simulink model "modelo_fisico_v18"  (R2021a)
settings: Solver=ode23  StartTime=0.0  StopTime=inf  MinStep=1e-4
values from neighbouring files (symbols this model uses):
  a_hMax = 0.75    [Datos_ProyectoGlobal_AyCD_Cantu_LagoTejo.m]    (also in Datos_v18.m; PID_calculado.mat)
  a_tMax = 0.8    [Datos_ProyectoGlobal_AyCD_Cantu_LagoTejo.m]    (also in Datos_v18.m; PID_calculado.mat)
  b_cx = 1e6    (= 1000000)    [Datos_ProyectoGlobal_AyCD_Cantu_LagoTejo.m]    (also in Datos_v18.m; PID_calculado.mat)
  b_cy = 1e7    (= 10000000)    [Datos_ProyectoGlobal_AyCD_Cantu_LagoTejo.m]    (also in Datos_v18.m; PID_calculado.mat)
  b_eq_h = ((b_hd + b_hm*(i_h^2))*2/(r_hd^2))    (= 31004.4444444)    [Datos_ProyectoGlobal_AyCD_Cantu_LagoTejo.m]    (also in Datos_v18.m; PID_calculado.mat)
  b_eq_t = ((b_td + b_tm*(i_t^2))/(r_td^2))    (= 21607.2)    [Datos_ProyectoGlobal_AyCD_Cantu_LagoTejo.m]    (also in Datos_v18.m; PID_calculado.mat)
  b_hb = 1e8    (= 100000000)    [Datos_ProyectoGlobal_AyCD_Cantu_LagoTejo.m]    (also in Datos_v18.m; PID_calculado.mat)
  b_hEb = 2.2e9    (= 2200000000)    [Datos_ProyectoGlobal_AyCD_Cantu_LagoTejo.m]    (also in Datos_v18.m; PID_calculado.mat)
  b_t = 90    [Datos_ProyectoGlobal_AyCD_Cantu_LagoTejo.m]    (also in Datos_v18.m; PID_calculado.mat)
  b_tb = 5e6    (= 5000000)    [Datos_ProyectoGlobal_AyCD_Cantu_LagoTejo.m]    (also in Datos_v18.m; PID_calculado.mat)
  b_tw = 3e3    (= 3000)    [Datos_ProyectoGlobal_AyCD_Cantu_LagoTejo.m]    (also in Datos_v18.m; PID_calculado.mat)
  b_wu = 150    [Datos_ProyectoGlobal_AyCD_Cantu_LagoTejo.m]    (also in Datos_v18.m; PID_calculado.mat)
  bah = M_eq_h*n_h*omega_h    [PID_Izaje_B.m]    (also in PID_calculado.mat = 387555.555556)
  bat = M_eq_t*n_t*omega_t    [PID_Carro_B.m]    (also in PID_calculado.mat = 270090)
  CI_h = 5    [Datos_ProyectoGlobal_AyCD_Cantu_LagoTejo.m]    (also in Datos_v18.m; PID_calculado.mat)
  CI_t = -16.25    [Datos_ProyectoGlobal_AyCD_Cantu_LagoTejo.m]    (also in Datos_v18.m; PID_calculado.mat)
  d_t = 1e-3    (= 0.001)    [Datos_ProyectoGlobal_AyCD_Cantu_LagoTejo.m]    (also in Datos_v18.m; PID_calculado.mat)
  g = 9.80665    [Datos_ProyectoGlobal_AyCD_Cantu_LagoTejo.m]    (also in Datos_v18.m; PID_calculado.mat)
  H_c = 2.5    [Datos_ProyectoGlobal_AyCD_Cantu_LagoTejo.m]    (also in Datos_v18.m; PID_calculado.mat)
  i_h = 22    [Datos_ProyectoGlobal_AyCD_Cantu_LagoTejo.m]    (also in Datos_v18.m; PID_calculado.mat)
  i_t = 30    [Datos_ProyectoGlobal_AyCD_Cantu_LagoTejo.m]    (also in Datos_v18.m; PID_calculado.mat)
  k_cy = 1.8e9    (= 1800000000)    [Datos_ProyectoGlobal_AyCD_Cantu_LagoTejo.m]    (also in Datos_v18.m; PID_calculado.mat)
  k_tw = 4.8e5    (= 480000)    [Datos_ProyectoGlobal_AyCD_Cantu_LagoTejo.m]    (also in Datos_v18.m; PID_calculado.mat)
  k_wu = 2.36e8    (= 236000000)    [Datos_ProyectoGlobal_AyCD_Cantu_LagoTejo.m]    (also in Datos_v18.m; PID_calculado.mat)
  Kd_bal = [-2.22044604925e-16 2.22044604925e-16 2.22044604925e-16 0 0 0 0 0 -2.22044604925e-16 0 2.22044604925e-16 -2.22044604925e-16 ... (296091 elements, 501x591)]    [Kp_Kd_balanceo.mat]    (also in PD_Balanceo.m = zeros(length(ML),length(L)))
  Kp_bal = [5.11381136401 5.1081388039 5.10248507909 5.09685008556 5.09123372013 5.08563588037 5.08005646467 5.07449537218 5.06895250283 5.06342775732 5.05792103709 5.05243224433 ... (296091 elements, 501x591)]    [Kp_Kd_balanceo.mat]    (also in PD_Balanceo.m = Kd_bal)
  ksah = M_eq_h*n_h*(omega_h^2)    [PID_Izaje_B.m]    (also in PID_calculado.mat = 922348.374575)
  ksat = M_eq_t*n_t*(omega_t^2)    [PID_Carro_B.m]    (also in PID_calculado.mat = 972648.108)
  ksiah = M_eq_h*n_h*(omega_h^3)    [PID_Izaje_B.m]    (also in PID_calculado.mat = 2195108.57705)
  ksiat = M_eq_t*n_t*(omega_t^3)    [PID_Carro_B.m]    (also in PID_calculado.mat = 3502700.36653)
  lim_xDer = 50    [Datos_ProyectoGlobal_AyCD_Cantu_LagoTejo.m]    (also in Datos_v18.m; PID_calculado.mat)
  lim_xDer_ult = 51    [Datos_ProyectoGlobal_AyCD_Cantu_LagoTejo.m]    (also in Datos_v18.m; PID_calculado.mat)
  lim_xIzq = -30    [Datos_ProyectoGlobal_AyCD_Cantu_LagoTejo.m]    (also in Datos_v18.m; PID_calculado.mat)
  lim_xIzq_ult = -31    [Datos_ProyectoGlobal_AyCD_Cantu_LagoTejo.m]    (also in Datos_v18.m; PID_calculado.mat)
  lim_yInf = -20    [Datos_ProyectoGlobal_AyCD_Cantu_LagoTejo.m]    (also in Datos_v18.m; PID_calculado.mat)
  lim_yInf_ult = -21    [Datos_ProyectoGlobal_AyCD_Cantu_LagoTejo.m]    (also in Datos_v18.m; PID_calculado.mat)
  lim_ySup = 40    [Datos_ProyectoGlobal_AyCD_Cantu_LagoTejo.m]    (also in Datos_v18.m; PID_calculado.mat)
  lim_ySup_ult = 41    [Datos_ProyectoGlobal_AyCD_Cantu_LagoTejo.m]    (also in Datos_v18.m; PID_calculado.mat)
  M_cMax = 50000    [Datos_ProyectoGlobal_AyCD_Cantu_LagoTejo.m]    (also in Datos_v18.m; PID_calculado.mat)
  M_cMin = 2000    [Datos_ProyectoGlobal_AyCD_Cantu_LagoTejo.m]    (also in Datos_v18.m; PID_calculado.mat)
  M_eq_h = (J_hd_hEb+J_hm_hb*i_h^2)*2/r_hd^2    (= 65137.7777778)    [Datos_ProyectoGlobal_AyCD_Cantu_LagoTejo.m]    (also in Datos_v18.m; PID_calculado.mat)
  M_eq_t = ((J_td + J_tm_tb*(i_t^2))/(r_td^2))    (= 30000)    [Datos_ProyectoGlobal_AyCD_Cantu_LagoTejo.m]    (also in Datos_v18.m; PID_calculado.mat)
  M_l_max = 32500    [Datos_ProyectoGlobal_AyCD_Cantu_LagoTejo.m]    (also in Datos_v18.m; PID_calculado.mat)
  M_l_nom = 65000    [Datos_ProyectoGlobal_AyCD_Cantu_LagoTejo.m]    (also in Datos_v18.m; PID_calculado.mat)
  M_s = 15000    [Datos_ProyectoGlobal_AyCD_Cantu_LagoTejo.m]    (also in Datos_v18.m; PID_calculado.mat)
  M_t = 30000    [Datos_ProyectoGlobal_AyCD_Cantu_LagoTejo.m]    (also in Datos_v18.m; PID_calculado.mat)
  P_h_nom = 956.15e3    (= 956150)    [Datos_ProyectoGlobal_AyCD_Cantu_LagoTejo.m]    (also in Datos_v18.m; PID_calculado.mat)
  r_hd = 0.75    [Datos_ProyectoGlobal_AyCD_Cantu_LagoTejo.m]    (also in Datos_v18.m; PID_calculado.mat)
  r_td = 0.5    [Datos_ProyectoGlobal_AyCD_Cantu_LagoTejo.m]    (also in Datos_v18.m; PID_calculado.mat)
  T_hbMax = 5e4    (= 50000)    [Datos_ProyectoGlobal_AyCD_Cantu_LagoTejo.m]    (also in Datos_v18.m; PID_calculado.mat)
  T_hEbMax = 1.1e6    (= 1100000)    [Datos_ProyectoGlobal_AyCD_Cantu_LagoTejo.m]    (also in Datos_v18.m; PID_calculado.mat)
  T_hmMax = 2e4    (= 20000)    [Datos_ProyectoGlobal_AyCD_Cantu_LagoTejo.m]    (also in Datos_v18.m; PID_calculado.mat)
  T_tbMax = 5e3    (= 5000)    [Datos_ProyectoGlobal_AyCD_Cantu_LagoTejo.m]    (also in Datos_v18.m; PID_calculado.mat)
  T_tmMax = 3e3    (= 3000)    [Datos_ProyectoGlobal_AyCD_Cantu_LagoTejo.m]    (also in Datos_v18.m; PID_calculado.mat)
  tau_hm = 1e-3    (= 0.001)    [Datos_ProyectoGlobal_AyCD_Cantu_LagoTejo.m]    (also in Datos_v18.m; PID_calculado.mat)
  tau_tm = 1e-3    (= 0.001)    [Datos_ProyectoGlobal_AyCD_Cantu_LagoTejo.m]    (also in Datos_v18.m; PID_calculado.mat)
  v_hMax_0 = 3    [Datos_ProyectoGlobal_AyCD_Cantu_LagoTejo.m]    (also in Datos_v18.m; PID_calculado.mat)
  v_hMax_l = 1.5    [Datos_ProyectoGlobal_AyCD_Cantu_LagoTejo.m]    (also in Datos_v18.m; PID_calculado.mat)
  v_tMax = 4    [Datos_ProyectoGlobal_AyCD_Cantu_LagoTejo.m]    (also in Datos_v18.m; PID_calculado.mat)
  xc = [-28.75 -26.25 -23.75 -21.25 -18.75 -16.25 -13.75 -11.25 -8.75 -6.25 -3.75 -1.25 ... (32 elements, 1x32)]    [PID_calculado.mat]    (also in Perfil_Carga.m = -30+1.25:2.5:50-1.25)
  Y_sb = 15    [Datos_ProyectoGlobal_AyCD_Cantu_LagoTejo.m]    (also in Datos_v18.m; PID_calculado.mat)
  Y_t0 = 45    [Datos_ProyectoGlobal_AyCD_Cantu_LagoTejo.m]    (also in Datos_v18.m; PID_calculado.mat)
  yc = [0 0 0 2.5 0 2.5 0 2.5 0 0 0 0 ... (32 elements, 1x32)]    [PID_calculado.mat]    (also in Perfil_Carga.m = yc2)
undefined symbols (not defined in the file or in its folder): bcx, bcy, Cond_Ini_h, Cond_Ini_t, Kcy
libraries: simulink x13
(part 1 of 3)
settings Model: SimulationMode=accelerator  Creator=Maxi  LastModifiedBy=maxim
settings SolverCC: InitialStep=1e-3  MaxConsecutiveZCs=10000  MaxConsecutiveMinStep=10000000  ZeroCrossAlgorithm=Adaptive  AlgebraicLoopSolver=TrustRegion
settings DebuggingCC: AlgebraicLoopMsg=none  MaskedZcDiagnostic=none  IgnoredZcDiagnostic=none  SFUnusedDataAndEventsDiag=none  UnderSpecifiedDimensionMsg=warning
settings RTWCC: DLArmComputeVersion=20.02.1

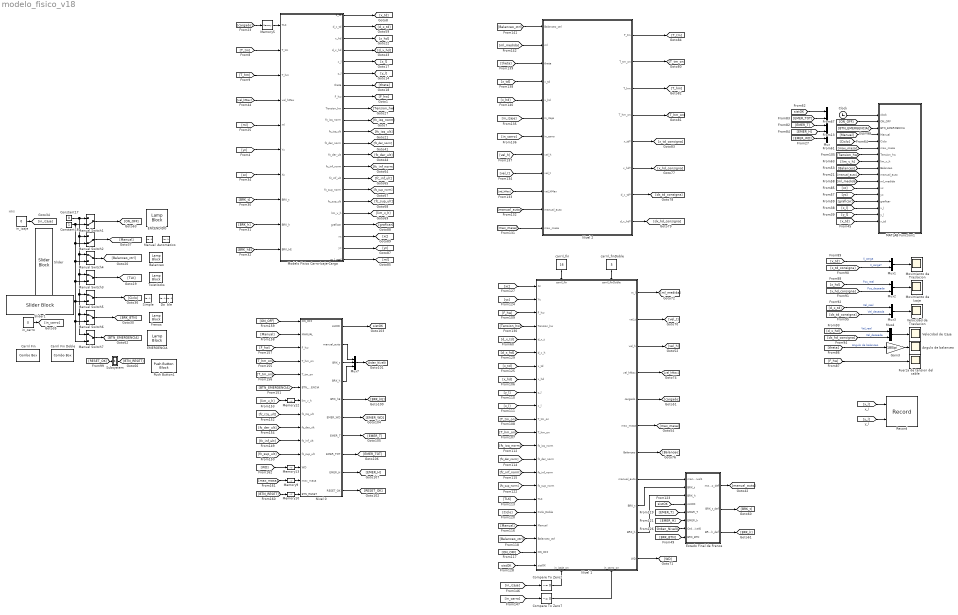
== system modelo_fisico_v18 ==
  note: HMI
  "  Do" : LampBlock  LabelPosition=Hide
  Angulo de balanceo : Scope
  Automático : LampBlock  LabelPosition=Hide
  Balanceo : LampBlock  LabelPosition=Hide
  Carril Fin : ComboBox  LabelPosition=Hide  SelectedLabel=16
      settings: Values={{'1', '2', '3', '4', '5', '6', '7', '8', '9', '10', '11', '12', '13', '14', '15', '16', '17', '18'}, [1 2 3 4 5 6 7 8 9 10 11 12 13 14 15 16 17 18]}
  Carril Fin Doble : ComboBox  LabelPosition=Hide  SelectedLabel=5
      settings: Values={{'1', '2', '3', '4', '5', '6', '7', '8', '9', '10', '11', '12', '13', '14', '15', '16', '17', '18'}, [1 2 3 4 5 6 7 8 9 10 11 12 13 14 15 16 17 18]}
  Clock : Clock
  Compare To Zero2 : simulink/Logic and Bit Operations/Compare To Zero  relop=~=  OutDataTypeStr=boolean
  Compare To Zero7 : simulink/Logic and Bit Operations/Compare To Zero  relop=~=  OutDataTypeStr=boolean
  Constant17 : Constant  Value=0
  Constant18 : Constant
  EMERGENCIA : LampBlock  LabelPosition=Hide
  ENCENDIDO : LampBlock  LabelPosition=Hide
  Estado Final de Frenos : Subsystem
  Frenos : LampBlock  LabelPosition=Hide
  Fuerza de tension del cable : Scope
  Gain3 : Gain  Gain=180/pi
  MATLAB Function1 : MATLAB Function  TreatAsAtomicUnit=on
  Manual : LampBlock  LabelPosition=Hide
  Manual Switch1 : ManualSwitch  CurrentSetting=0
  Manual Switch2 : ManualSwitch  CurrentSetting=0
  Manual Switch{3..7} (5 alike) : ManualSwitch
  Memory{5,9..10,12..13} (5 alike) : Memory
  Modelo Fisico Carro-Izaje-Carga : Subsystem
  Movimiento de Izaje : Scope
  Movimiento de Traslacion : Scope
  Mux : Mux  Inputs=5
  Mux{1..4} (4 alike) : Mux  Inputs=2
  Mux7 : Mux  Inputs=3
  Nivel 0 : Stateflow chart  TreatAsAtomicUnit=on
      settings: PortSchema="{\"entries\":[{\"content\":{\"sides\":[{\"content\":{\"connectorIds\":[\"In6\",\"In7\",\"In5\",\"In2\",\"In1\",\"In3\",\"In4\",\"In8\",\"In9\",\"In10\",\"In11\",\"In12\",\"In13\",\"In14\"]},\"type\":\"ConnectorPlacement.EquallySpacedRectSide\",\"uuid\":\"e3679c49-321c-4245-9f4d-6b72d70eef8d\"},{\"content\":{\"connectorIds\":[\"Out1\",\"Out3\",\"Out5\",\"Out4\",\"Out2\",\"Out6\",\"Out7\",\"Out8\",\"Out9\",\"Out10\"],\"side\":\"RIGHT\"},\"type\":\"ConnectorPlacement.EquallySpacedRectSide\",\"uuid\":\"16418e5e-e28d-455d-933a-43b8d78ab460\"},{\"content\":{\"side\":\"TOP\"},\"type\":\"ConnectorPlacement.EquallySpacedRectSide\",\"uuid\":\"c85d7e80-ad5f-4217-ba10-6288ee566bb8\"}]},\"type\":\"ConnectorPlacement.EquallySpacedConnector\",\"uuid\":\"c38c6e76-5322-4b57-8473-560e5b1141d3\"}],\"packageUris\":[\"http://schema.mathworks.com/mf0/Connector/R2020b\"],\"version\":\"1.0\"}"
  Nivel 1 : Stateflow chart  TreatAsAtomicUnit=on
      settings: PortSchema="{\"entries\":[{\"content\":{\"sides\":[{\"content\":{\"connectorIds\":[\"In23\",\"In22\",\"In12\",\"In24\",\"In21\",\"In20\",\"In10\",\"In11\",\"In19\",\"In5\",\"In9\",\"In4\",\"In15\",\"In16\",\"In17\",\"In18\",\"In3\",\"In14\",\"In13\",\"In6\",\"In7\",\"In8\"]},\"type\":\"ConnectorPlacement.EquallySpacedRectSide\",\"uuid\":\"68c99711-1ca5-49d6-a421-ad202abad7a3\"},{\"content\":{\"connectorIds\":[\"Out5\",\"Out8\",\"Out6\",\"Out7\",\"Out9\",\"Out11\",\"Out2\",\"Out3\",\"Out4\",\"Out1\",\"Out10\"],\"side\":\"RIGHT\"},\"type\":\"ConnectorPlacement.EquallySpacedRectSide\",\"uuid\":\"bc0f262a-18b8-4d7b-9b7f-403e0cd3788b\"},{\"content\":{\"connectorIds\":[\"In25\",\"In26\"],\"side\":\"TOP\"},\"type\":\"ConnectorPlacement.EquallySpacedRectSide\",\"uuid\":\"2d69c358-e680-43cc-a1d0-9fcf2b39de17\"},{\"content\":{\"connectorIds\":[\"In1\",\"In2\"],\"side\":\"BOTTOM\"},\"type\":\"ConnectorPlacement.EquallySpacedRectSide\",\"uuid\":\"d4a5b5d0-6661-40f6-8d98-5cae5bd8c928\"}]},\"type\":\"ConnectorPlacement.EquallySpacedConnector\",\"uuid\":\"d3c5d26b-109c-4d02-96fa-92f2f1f71ce2\"}],\"packageUris\":[\"http://schema.mathworks.com/mf0/Connector/R2020b\"],\"version\":\"1.0\"}"
  Nivel 2 : Subsystem
  Push Button1 : PushButtonBlock  ButtonText=RESET
  Record : Record  FileSettingsInternal="{\"entries\":[{\"content\":{\"excelSettings\":{\"content\":{},\"type\":\"Streamout.ExcelSettings\"}},\"type\":\"Streamout.FileSettingStorage\",\"uuid\":\"e8508c65-0194-4cdc-8554-125005728cb5\"}],\"packageUris\":[\"http://schema.mathworks.com/mf0/streamout_blocks/R2020a\"],\"version\":\"1.0\"}"  Layout=[1 1]  SignalsInternal="{\"entries\":[{\"content\":{\"signals\":[{\"content\":{\"blockPath\":[\"modelo_fisico_v18/Record\"],\"channel\":[],\"dimensions\":[1],\"domain\":\"modelo_fisico_v18/record\",\"lineColor\":\"#edb120\",\"plots\":[1],\"port\":1,\"sid\":[\"\"],\"signalID\":255712,\"signalName\":\"x_l\"},\"type\":\"RecordBlkView.Signal\",\"uuid\":\"63b07128-c455-47b4-8ee9-e193b57c47c9\"},{\"content\":{\"blockPath\":[\"modelo_fisico_v18/Record\"],\"channel\":[],\"dimensions\":[1],\"domain\":\"modelo_fisico_v18/record\",\"lineColor\":\"#7e2f8e\",\"plots\":[1],\"port\":2,\"sid\":[\"\"],\"signalID\":255716,\"signalName\":\"y_l\"},\"type\":\"RecordBlkView.Signal\",\"uuid\":\"f3964feb-c2bd-47d9-a82e-f0022fb4662f\"}]},\"type\":\"RecordBlkView.InputSignals\",\"uuid\":\"bfb33c13-72dd-4754-b344-f1860909a54a\"}],\"packageUris\":[\"http://schema.mathworks.com/mf0/streamout_blocks/R2020a\"],\"version\":\"1.0\"}"  VisualizationBindings="{\"xyplotplugin\":{\"info\":[{\"series\":[{\"bindingParametersList\":[{\"parameter\":\"X-Axis\",\"signalID\":255712,\"signalName\":\"x_l\"},{\"parameter\":\"Y-Axis\",\"signalID\":255716,\"signalName\":\"y_l\"}],\"seriesID\":213},{\"bindingParametersList\":[],\"seriesID\":320},{\"bindingParametersList\":[],\"seriesID\":767},{\"bindingParametersList\":[],\"seriesID\":639}],\"subplotID\":1}]}}"
  Simple : LampBlock  LabelPosition=Hide
  Slider : SliderBlock  ScaleMin=-3  ScaleMax=3  TickInterval=1
  Slider1 : SliderBlock  ScaleMin=-4  ScaleMax=+4  TickInterval=1
  Subsystem : Subsystem
  Twistlocks : LampBlock  LabelPosition=Hide
  Velocidad de Izaje : Scope
  Velocidad de Traslacion : Scope
  "ble   " : LampBlock  LabelPosition=Hide
  carril_fin : Constant  Value=16
  carril_finDoble : Constant  Value=5
  in_carro : Constant  Value=0
  in_izaje : Constant  Value=0
  tag scope: Orden_Nivel0=global, sistOK=global
  wires:
  Modelo Fisico Carro-Izaje-Carga/1(x_td) -> [x_td]
  Modelo Fisico Carro-Izaje-Carga/3(x_hd) -> [x_hd]
  Modelo Fisico Carro-Izaje-Carga/7(theta) -> [theta]
  [yc] -> Modelo Fisico Carro-Izaje-Carga/6(Yc)
  Modelo Fisico Carro-Izaje-Carga/5(x_l) -> [x_l]
  Modelo Fisico Carro-Izaje-Carga/6(y_l) -> [y_l]
  Modelo Fisico Carro-Izaje-Carga/8(F_hw) -> [F_hw]
  Modelo Fisico Carro-Izaje-Carga/2(d_x_td) -> [d_x_td]
  Modelo Fisico Carro-Izaje-Carga/4(d_x_hd) -> [d_x_hd]
  [T_tm] -> Modelo Fisico Carro-Izaje-Carga/2(T_tm)
  [T_hm] -> Modelo Fisico Carro-Izaje-Carga/3(T_hm)
  [ml] -> Modelo Fisico Carro-Izaje-Carga/5(ml)
  [sistOK] -> Mux/1
  [EMER_TOT] -> Mux/2
  [EMER_T] -> Mux/3
  [EMER_H] -> Mux/4
  [EMER_WD] -> Mux/5
  [theta] -> Gain3/1  "Angulo de balanceo"
  [F_hw] -> Fuerza de tension del cable/1
  [dx_hd_consigna] -> Mux4/2  "Vel_deseada"
  [d_x_td] -> Mux3/1  "Vel_real"
  [x_hd_consigna] -> Mux2/2  "Pos_deseada"
  Mux2/1 -> Movimiento de Izaje/1
  Mux4/1 -> Velocidad de Izaje/1
  [d_x_hd] -> Mux4/1  "Vel_real"
  [x_td] -> Mux1/1  "X_carga"
  Mux3/1 -> Velocidad de Traslacion/1
  [x_td_consigna] -> Mux1/2  "X_carga*"
  [x_hd] -> Mux2/1  "Pos_real"
  Mux1/1 -> Movimiento de Traslacion/1
  [dx_td_consigna] -> Mux3/2  "Vel_deseada"
  Gain3/1 -> Angulo de balanceo/1
  [BRK_h] -> Modelo Fisico Carro-Izaje-Carga/9(BRK_h)
  [BRK_hE] -> Modelo Fisico Carro-Izaje-Carga/10(BRK_hE)
  [BRK_t] -> Modelo Fisico Carro-Izaje-Carga/8(BRK_t)
  Modelo Fisico Carro-Izaje-Carga/15(fc_inf_ult) -> [fc_inf_ult]
  Modelo Fisico Carro-Izaje-Carga/18(lim_v_h) -> [lim_v_h]
  [cargado] -> Memory5/1
  Memory5/1 -> Modelo Fisico Carro-Izaje-Carga/1(TLK)
  Modelo Fisico Carro-Izaje-Carga/14(fc_inf_norm) -> [fc_inf_norm]
  Modelo Fisico Carro-Izaje-Carga/17(fc_sup_ult) -> [fc_sup_ult]
  Modelo Fisico Carro-Izaje-Carga/13(fc_der_ult) -> [fc_der_ult]
  Modelo Fisico Carro-Izaje-Carga/10(fc_izq_norm) -> [fc_izq_norm]
  Modelo Fisico Carro-Izaje-Carga/11(fc_izq_ult) -> [fc_izq_ult]
  Modelo Fisico Carro-Izaje-Carga/12(fc_der_norm) -> [fc_der_norm]
  Modelo Fisico Carro-Izaje-Carga/16(fc_sup_norm) -> [fc_sup_norm]
  [xc] -> Modelo Fisico Carro-Izaje-Carga/7(Xc)
  [vel_hMax] -> Modelo Fisico Carro-Izaje-Carga/4(vel_hMax)
  [x_l] -> Record/1
  [y_l] -> Record/2
  Modelo Fisico Carro-Izaje-Carga/9(Tension_hw) -> [Tension_hw]
  Estado Final de Frenos/2(BRK_t_def) -> [BRK_t]
  [EMER_H] -> Estado Final de Frenos/6(EMER_h)
  [fc_inf_norm] -> Nivel 1/17(fc_inf_norm)
  [Orden_Nivel0] -> Estado Final de Frenos/7(Orden_Nivel0)
  [T_tm_on] -> Nivel 1/9(T_tm_on)
  Estado Final de Frenos/3(BRK_h_def) -> [BRK_h]
  [sistOK] -> Nivel 1/8(sistOK)
  Nivel 1/10(WD) -> [WD]
  [fc_der_norm] -> Nivel 1/16(fc_der_norm)
  Nivel 1/3(manual_auto) -> Estado Final de Frenos/1(manual_auto_Nivel1)
  [EMER_T] -> Estado Final de Frenos/5(EMER_T)
  [ON_OFF] -> Nivel 1/7(ON_OFF)
  Nivel 1/7(vel_hMax) -> [vel_hMax]
  carril_fin/1 -> Nivel 1/25(carril_fin)
  [d_x_hd] -> Nivel 1/20(d_x_h)
  [x_td] -> Nivel 1/10(x_td)
  [F_hw] -> Nivel 1/12(F_hw)
  Nivel 1/1(BRK_h) -> Estado Final de Frenos/3(BRK_h)
  [fc_izq_norm] -> Nivel 1/15(fc_izq_norm)
  Nivel 1/9(cargado) -> [cargado]
  [TLK] -> Nivel 1/3(TLK)
  [sistOK] -> Estado Final de Frenos/4(sistOK)
  [d_x_td] -> Nivel 1/21(d_x_t)
  [Ciclo] -> Nivel 1/14(Ciclo_Doble)
  Estado Final de Frenos/1(manual_auto_def) -> [manual_auto]
  Nivel 1/4(BRK_t) -> Estado Final de Frenos/2(BRK_t)
  [Manual] -> Nivel 1/13(Manual)
  [Balanceo_ctrl] -> Nivel 1/6(Balanceo_ctrl)
  Nivel 1/2(Balanceo) -> [Balanceo]
  [x_hd] -> Nivel 1/11(x_hd)
  [xc] -> Nivel 1/23(Xc)
  [yc] -> Nivel 1/22(Yc)
  Nivel 1/5(m_l) -> [ml_medida]
  [fc_sup_norm] -> Nivel 1/18(fc_sup_norm)
  [y_l] -> Nivel 1/19(y_l)
  [x_l] -> Nivel 1/5(x_l)
  Nivel 1/6(vel_h) -> [vel_h]
  [T_hm_on] -> Nivel 1/4(T_hm_on)
  Nivel 1/8(vel_t) -> [vel_t]
  carril_finDoble/1 -> Nivel 1/26(carril_finDoble)
  [Tension_hw] -> Nivel 1/24(Tension_hw)
  [ml_medida] -> Nivel 2/2(ml)
  [x_hd] -> Nivel 2/5(x_hd)
  Nivel 2/5(x_td*) -> [x_td_consigna]
  Nivel 2/2(T_tm_on) -> [T_tm_on]
  Nivel 2/4(T_hm_on) -> [T_hm_on]
  [Balanceo_ctrl] -> Nivel 2/1(Balanceo_ctrl)
  Nivel 2/6(x_hd*) -> [x_hd_consigna]
  Nivel 2/8(d_x_hd*) -> [dx_hd_consigna]
  Nivel 2/1(T_tm) -> [T_tm]
  Nivel 2/3(T_hm) -> [T_hm]
  [vel_h] -> Nivel 2/8(vel_h)
  [x_td] -> Nivel 2/4(x_td)
  [in_izaje] -> Nivel 2/6(in_izaje)
  Nivel 2/7(d_x_td*) -> [dx_td_consigna]
  [theta] -> Nivel 2/3(theta)
  [vel_hMax] -> Nivel 2/10(vel_hMax)
  [in_carro] -> Nivel 2/7(in_carro)
  [max_masa] -> Nivel 2/12(max_masa)
  [manual_auto] -> Nivel 2/11(manual_auto)
  [vel_t] -> Nivel 2/9(vel_t)
  Compare To Zero7/1 -> Nivel 1/2(in_carro_on)
  [in_carro] -> Compare To Zero7/1
  Compare To Zero2/1 -> Nivel 1/1(in_izaje_on)
  [in_izaje] -> Compare To Zero2/1
  [max_masa] -> Memory9/1
  [T_tm_on] -> Nivel 0/1(T_tm_on)
  Nivel 0/10(RESET_OK) -> [RESET_OK]
  [T_hm_on] -> Nivel 0/2(T_hm_on)
  [fc_izq_ult] -> Nivel 0/8(fc_izq_ult)
  Mux7/1 -> [Orden_Nivel0]
  Nivel 0/5(BRK_t) -> Mux7/2
  [Manual] -> Nivel 0/7(MANUAL)
  [ON_OFF] -> Nivel 0/6(ON_OFF)
  Nivel 0/9(EMER_H) -> [EMER_H]
  [lim_v_h] -> Memory12/1
  [BTN_RESET] -> Memory10/1
  [fc_der_ult] -> Nivel 0/9(fc_der_ult)
  Nivel 0/1(sistOK) -> [sistOK]
  Nivel 0/8(EMER_TOT) -> [EMER_TOT]
  Nivel 0/4(BRK_h) -> Mux7/3
  [BTN_EMERGENCIA] -> Nivel 0/3(BTN_EMERGENCIA)
  Memory12/1 -> Nivel 0/4(lim_v_h)
  Memory13/1 -> Nivel 0/12(WD)
  Nivel 0/3(manual_auto) -> Mux7/1
  Nivel 0/7(EMER_T) -> [EMER_T]
  [WD] -> Memory13/1
  Nivel 0/6(EMER_WD) -> [EMER_WD]
  [fc_inf_ult] -> Nivel 0/10(fc_inf_ult)
  Nivel 0/2(BRK_hE) -> [BRK_hE]
  [F_hw] -> Nivel 0/5(F_hw)
  [fc_sup_ult] -> Nivel 0/11(fc_sup_ult)
  Modelo Fisico Carro-Izaje-Carga/19(graficar) -> [graficar]
  Modelo Fisico Carro-Izaje-Carga/20(xc) -> [xc]
  Modelo Fisico Carro-Izaje-Carga/21(yc) -> [yc]
  Modelo Fisico Carro-Izaje-Carga/22(m_l_real) -> [ml]
  Nivel 1/11(max_masa) -> [max_masa]
  Memory9/1 -> Nivel 0/13(max_masa)
  Memory10/1 -> Nivel 0/14(BTN_RESET)
  Constant18/1 -> Manual Switch2/2, Manual Switch4/2, Manual Switch3/2, Manual Switch6/2, Manual Switch7/2, Manual Switch5/2, Manual Switch1/2
  Manual Switch4/1 -> [Balanceo_ctrl]
  in_carro/1 -> [in_carro]
  Manual Switch6/1 -> [BRK_BTN]
  Constant17/1 -> Manual Switch2/1, Manual Switch4/1, Manual Switch3/1, Manual Switch6/1, Manual Switch7/1, Manual Switch5/1, Manual Switch1/1
  Manual Switch1/1 -> [ON_OFF]
  Manual Switch5/1 -> [Ciclo]
  in_izaje/1 -> [in_izaje]
  Manual Switch3/1 -> [TLK]
  Subsystem/1(Out1) -> [BTN_RESET]
  Manual Switch2/1 -> [Manual]
  [RESET_OK] -> Subsystem/1(" ")
  Manual Switch7/1 -> [BTN_EMERGENCIA]
  [BRK_BTN] -> Estado Final de Frenos/8(BRK_BTN)
  Clock/1 -> MATLAB Function1/1(clock)
  [ON_OFF] -> MATLAB Function1/2(ON_OFF)
  [BTN_EMERGENCIA] -> MATLAB Function1/3(BTN_EMERGENCIA)
  [Manual] -> MATLAB Function1/4(Manual)
  [Ciclo] -> MATLAB Function1/5(Ciclo)
  [max_masa] -> MATLAB Function1/6(max_masa)
  [Tension_hw] -> MATLAB Function1/7(Tension_hw)
  [lim_v_h] -> MATLAB Function1/8(lim_v_h)
  [Balanceo] -> MATLAB Function1/9(Balanceo)
  [manual_auto] -> MATLAB Function1/10(manual_auto)
  [ml_medida] -> MATLAB Function1/11(ml_medida)
  [xc] -> MATLAB Function1/12(xc)
  [yc] -> MATLAB Function1/13(yc)
  [graficar] -> MATLAB Function1/14(graficar)
  [x_l] -> MATLAB Function1/15(x_l)
  [y_l] -> MATLAB Function1/16(y_l)
  [x_td] -> MATLAB Function1/17(x_td)

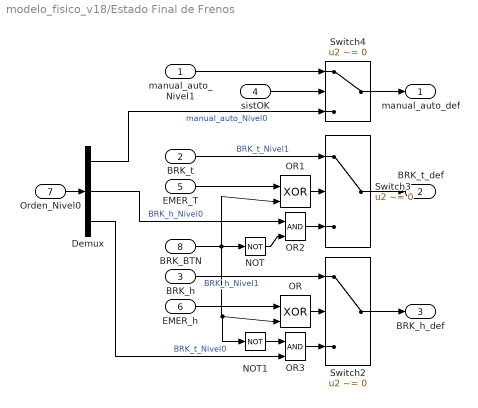
== system modelo_fisico_v18/Estado Final de Frenos ==
  manual_auto_Nivel1 : Inport
  BRK_t : Inport  Port=2
  BRK_h : Inport  Port=3
  sistOK : Inport  Port=4
  EMER_T : Inport  Port=5
  EMER_h : Inport  Port=6
  Orden_Nivel0 : Inport  Port=7
  BRK_BTN : Inport  Port=8
  Demux : Demux  Outputs=3
  NOT : Logic  Operator=NOT  IconShape=distinctive  AllPortsSameDT=off  OutDataTypeStr=boolean
  NOT1 : Logic  Operator=NOT  IconShape=distinctive  AllPortsSameDT=off  OutDataTypeStr=boolean
  OR : Logic  Operator=XOR  IconShape=distinctive  AllPortsSameDT=off  OutDataTypeStr=boolean
  OR1 : Logic  Operator=XOR  IconShape=distinctive  AllPortsSameDT=off  OutDataTypeStr=boolean
  OR2 : Logic  IconShape=distinctive  AllPortsSameDT=off  OutDataTypeStr=boolean
  OR3 : Logic  IconShape=distinctive  AllPortsSameDT=off  OutDataTypeStr=boolean
  Switch2 : Switch  Criteria=u2 ~= 0
  Switch3 : Switch  Criteria=u2 ~= 0
  Switch4 : Switch  Criteria=u2 ~= 0
  manual_auto_def : Outport
  BRK_t_def : Outport  Port=2
  BRK_h_def : Outport  Port=3
  wires:
  Switch3/1 -> BRK_t_def/1
  Switch2/1 -> BRK_h_def/1
  Switch4/1 -> manual_auto_def/1
  sistOK/1 -> Switch4/2
  BRK_t/1 -> Switch3/1  "BRK_t_Nivel1"
  BRK_h/1 -> Switch2/1  "BRK_h_Nivel1"
  manual_auto_Nivel1/1 -> Switch4/1
  Demux/2 -> OR2/1  "BRK_h_Nivel0"
  Demux/3 -> OR3/2  "BRK_t_Nivel0"
  Orden_Nivel0/1 -> Demux/1
  Demux/1 -> Switch4/3  "manual_auto_Nivel0"
  OR/1 -> Switch2/2
  EMER_T/1 -> OR1/1
  OR1/1 -> Switch3/2
  BRK_BTN/1 -> OR1/2, NOT/1, NOT1/1, OR/2
  OR2/1 -> Switch3/3
  NOT/1 -> OR2/2
  EMER_h/1 -> OR/1
  OR3/1 -> Switch2/3
  NOT1/1 -> OR3/1

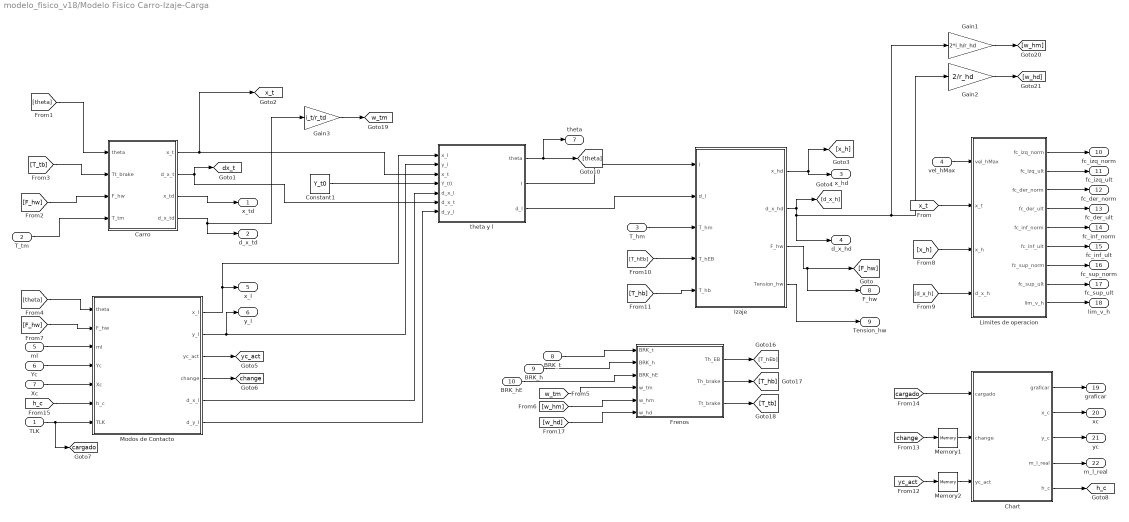
== system modelo_fisico_v18/Modelo Fisico Carro-Izaje-Carga ==
  TLK : Inport
  T_tm : Inport  Port=2
  T_hm : Inport  Port=3
  vel_hMax : Inport  Port=4
  ml : Inport  Port=5
  Yc : Inport  Port=6
  Xc : Inport  Port=7
  BRK_t : Inport  Port=8
  BRK_h : Inport  Port=9
  BRK_hE : Inport  Port=10
  Carro : Subsystem
  Chart : Stateflow chart  TreatAsAtomicUnit=on
      settings: PortSchema="{\"entries\":[{\"content\":{\"sides\":[{\"content\":{\"connectorIds\":[\"In1\",\"In2\",\"In3\"]},\"type\":\"ConnectorPlacement.EquallySpacedRectSide\",\"uuid\":\"3e82a7c2-bf75-4f61-8ed8-4dc94ac63b2a\"},{\"content\":{\"connectorIds\":[\"Out3\",\"Out4\",\"Out2\",\"Out5\",\"Out1\"],\"side\":\"RIGHT\"},\"type\":\"ConnectorPlacement.EquallySpacedRectSide\",\"uuid\":\"3bda0d7b-f5b8-4b7e-98a5-641e146bfa09\"},{\"content\":{\"connectorIds\":[],\"side\":\"TOP\"},\"type\":\"ConnectorPlacement.EquallySpacedRectSide\",\"uuid\":\"53c96370-adb7-4c5f-b84b-b565cd95f057\"}]},\"type\":\"ConnectorPlacement.EquallySpacedConnector\",\"uuid\":\"5926f053-77e4-4d2a-97aa-9f275575c8db\"}],\"packageUris\":[\"http://schema.mathworks.com/mf0/Connector/R2020b\"],\"version\":\"1.0\"}"
  Constant1 : Constant  Value=Y_t0
  Frenos : Subsystem
  Gain1 : Gain  Gain=2*i_h/r_hd
  Gain2 : Gain  Gain=2/r_hd
  Gain3 : Gain  Gain=i_t/r_td
  Izaje : Subsystem
  Limites de operacion : Subsystem
  Memory1 : Memory
  Memory2 : Memory
  Modos de Contacto : Subsystem
  theta y l : Subsystem
  x_td : Outport
  d_x_td : Outport  Port=2
  x_hd : Outport  Port=3
  d_x_hd : Outport  Port=4
  x_l : Outport  Port=5
  y_l : Outport  Port=6
  theta : Outport  Port=7
  F_hw : Outport  Port=8
  Tension_hw : Outport  Port=9
  fc_izq_norm : Outport  Port=10
  fc_izq_ult : Outport  Port=11
  fc_der_norm : Outport  Port=12
  fc_der_ult : Outport  Port=13
  fc_inf_norm : Outport  Port=14
  fc_inf_ult : Outport  Port=15
  fc_sup_norm : Outport  Port=16
  fc_sup_ult : Outport  Port=17
  lim_v_h : Outport  Port=18
  graficar : Outport  Port=19
  xc : Outport  Port=20
  yc : Outport  Port=21
  m_l_real : Outport  Port=22
  tag scope: cargado=global, change=global, dx_t=global, h_c=global, w_tm=global, x_t=global, yc_act=global
  wires:
  BRK_h/1 -> Frenos/2(BRK_h)
  BRK_t/1 -> Frenos/1(BRK_t)
  BRK_hE/1 -> Frenos/3(BRK_hE)
  [w_tm] -> Frenos/4(w_tm)
  [w_hm] -> Frenos/5(w_hm)
  Limites de operacion/2(fc_izq_ult) -> fc_izq_ult/1
  Limites de operacion/1(fc_izq_norm) -> fc_izq_norm/1
  Limites de operacion/6(fc_inf_ult) -> fc_inf_ult/1
  Gain2/1 -> [w_hd]
  Limites de operacion/9(lim_v_h) -> lim_v_h/1
  Limites de operacion/3(fc_der_norm) -> fc_der_norm/1
  Limites de operacion/4(fc_der_ult) -> fc_der_ult/1
  Limites de operacion/5(fc_inf_norm) -> fc_inf_norm/1
  Limites de operacion/7(fc_sup_norm) -> fc_sup_norm/1
  Gain3/1 -> [w_tm]
  vel_hMax/1 -> Limites de operacion/1(vel_hMax)
  Limites de operacion/8(fc_sup_ult) -> fc_sup_ult/1
  Gain1/1 -> [w_hm]
  Frenos/1(Th_EB) -> [T_hEb]
  Frenos/2(Th_brake) -> [T_hb]
  Frenos/3(Tt_brake) -> [T_tb]
  [w_hd] -> Frenos/6(w_hd)
  [theta] -> Carro/1(theta)
  [T_tb] -> Carro/2(Tt_brake)
  [F_hw] -> Carro/3(F_hw)
  T_tm/1 -> Carro/4(T_tm)
  Carro/2(d_x_t) -> theta y l/6(d_x_t), [dx_t]
  Carro/3(x_td) -> x_td/1
  Carro/4(d_x_td) -> Gain3/1, d_x_td/1
  Modos de Contacto/1(x_l) -> x_l/1, theta y l/1(x_l)
  Carro/1(x_t) -> [x_t], theta y l/3(x_t)
  Modos de Contacto/2(y_l) -> y_l/1, theta y l/2(y_l)
  theta y l/1(theta) -> [theta], theta/1
  Constant1/1 -> theta y l/4(Y_t0)
  Modos de Contacto/5(d_x_l) -> theta y l/5(d_x_l)
  Modos de Contacto/6(d_y_l) -> theta y l/7(d_y_l)
  [theta] -> Modos de Contacto/1(theta)
  [F_hw] -> Modos de Contacto/2(F_hw)
  ml/1 -> Modos de Contacto/3(ml)
  [h_c] -> Modos de Contacto/6(h_c)
  Yc/1 -> Modos de Contacto/4(Yc)
  Xc/1 -> Modos de Contacto/5(Xc)
  Modos de Contacto/4(change) -> [change]
  [T_hEb] -> Izaje/4(T_hEB)
  T_hm/1 -> Izaje/3(T_hm)
  [T_hb] -> Izaje/5(T_hb)
  theta y l/2(l) -> Izaje/1(l)
  theta y l/3(d_l) -> Izaje/2(d_l)
  Izaje/3(F_hw) -> F_hw/1, [F_hw]
  Izaje/1(x_hd) -> x_hd/1, [x_h]
  Izaje/2(d_x_hd) -> d_x_hd/1, Gain2/1, Gain1/1, [d_x_h]
  [x_t] -> Limites de operacion/2(x_t)
  [x_h] -> Limites de operacion/3(x_h)
  [d_x_h] -> Limites de operacion/4(d_x_h)
  Izaje/4(Tension_hw) -> Tension_hw/1
  [change] -> Memory1/1
  Chart/1(h_c) -> [h_c]
  Chart/4(x_c) -> xc/1
  Chart/3(graficar) -> graficar/1
  Chart/2(y_c) -> yc/1
  [yc_act] -> Memory2/1
  Modos de Contacto/3(yc_act) -> [yc_act]
  TLK/1 -> [cargado], Modos de Contacto/7(TLK)
  [cargado] -> Chart/1(cargado)
  Memory1/1 -> Chart/2(change)
  Memory2/1 -> Chart/3(yc_act)
  Chart/5(m_l_real) -> m_l_real/1

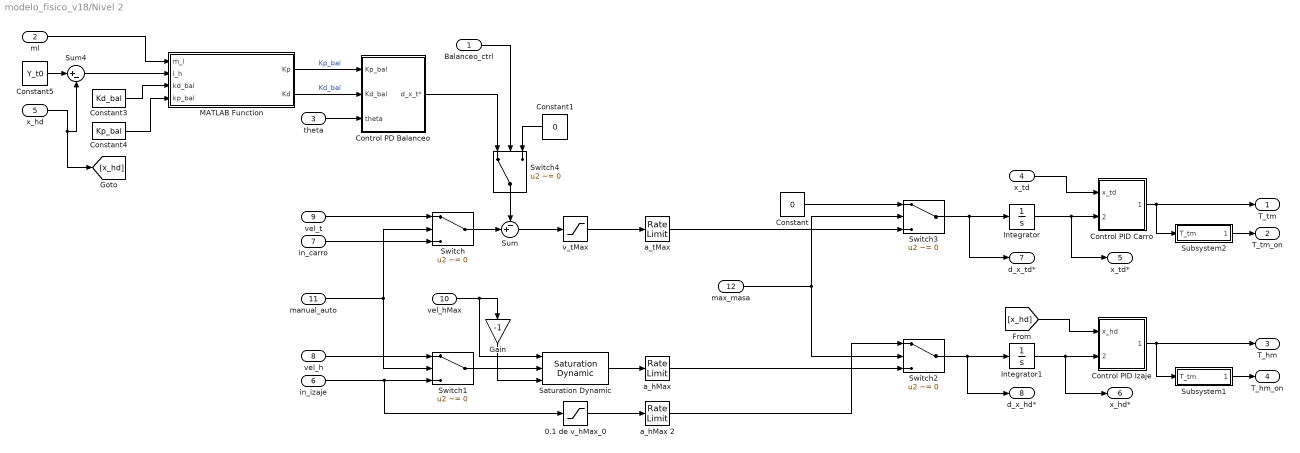
== system modelo_fisico_v18/Nivel 2 ==
  Balanceo_ctrl : Inport
  ml : Inport  Port=2
  theta : Inport  Port=3
  x_td : Inport  Port=4
  x_hd : Inport  Port=5
  in_izaje : Inport  Port=6
  in_carro : Inport  Port=7
  vel_h : Inport  Port=8
  vel_t : Inport  Port=9
  vel_hMax : Inport  Port=10
  manual_auto : Inport  Port=11
  max_masa : Inport  Port=12
  0.1 de v_hMax_0 : Saturate  UpperLimit=0  LowerLimit=-0.1*v_hMax_0
  Constant : Constant  Value=0
  Constant1 : Constant  Value=0
  Constant3 : Constant  Value=Kd_bal
  Constant4 : Constant  Value=Kp_bal
  Constant5 : Constant  Value=Y_t0
  Control PD Balanceo : Subsystem
  Control PID Carro : Subsystem
  Control PID Izaje : Subsystem
  Gain : Gain  Gain=-1
  Integrator : Integrator  InitialCondition=CI_t
  Integrator1 : Integrator  InitialCondition=CI_h
  MATLAB Function : MATLAB Function  TreatAsAtomicUnit=on
  Saturation Dynamic : simulink/Discontinuities/Saturation Dynamic  OutMin=[]  OutMax=[]  OutDataTypeStr=Inherit: Same as second input  OutDataType=fixdt(1, 16)  OutScaling=2^-10  DoSatur=off
  Subsystem1 : Subsystem
  Subsystem2 : Subsystem
  Sum : Sum  Inputs=-+|
  Sum4 : Sum  Inputs=|+-
  Switch{,1..4} (5 alike) : Switch  Criteria=u2 ~= 0
  a_hMax : RateLimiter  RisingSlewLimit=a_hMax  FallingSlewLimit=-a_hMax  SampleTimeMode=inherited
  a_hMax 2 : RateLimiter  RisingSlewLimit=a_hMax  FallingSlewLimit=-a_hMax  SampleTimeMode=inherited
  a_tMax : RateLimiter  RisingSlewLimit=a_tMax  FallingSlewLimit=-a_tMax  SampleTimeMode=inherited
  v_tMax : Saturate  UpperLimit=v_tMax  LowerLimit=-v_tMax
  T_tm : Outport
  T_tm_on : Outport  Port=2
  T_hm : Outport  Port=3
  T_hm_on : Outport  Port=4
  x_td* : Outport  Port=5
  x_hd* : Outport  Port=6
  d_x_td* : Outport  Port=7
  d_x_hd* : Outport  Port=8
  wires:
  manual_auto/1 -> Switch/2, Switch1/2
  Switch1/1 -> Saturation Dynamic/2
  vel_hMax/1 -> Saturation Dynamic/1, Gain/1
  Gain/1 -> Saturation Dynamic/3
  in_carro/1 -> Switch/3
  vel_h/1 -> Switch1/1
  Saturation Dynamic/1 -> a_hMax/1
  v_tMax/1 -> a_tMax/1
  Constant/1 -> Switch3/1
  0.1 de v_hMax_0/1 -> a_hMax 2/1
  vel_t/1 -> Switch/1
  Switch/1 -> Sum/2
  in_izaje/1 -> 0.1 de v_hMax_0/1, Switch1/3
  max_masa/1 -> Switch2/2, Switch3/2
  a_hMax 2/1 -> Switch2/1
  Sum/1 -> v_tMax/1
  a_tMax/1 -> Switch3/3
  a_hMax/1 -> Switch2/3
  Constant3/1 -> MATLAB Function/3(kd_bal)
  Balanceo_ctrl/1 -> Switch4/2
  Constant4/1 -> MATLAB Function/4(kp_bal)
  Constant5/1 -> Sum4/1
  x_hd/1 -> [x_hd], Sum4/2
  Sum4/1 -> MATLAB Function/2(l_h)
  ml/1 -> MATLAB Function/1(m_l)
  Constant1/1 -> Switch4/3
  MATLAB Function/1(Kp) -> Control PD Balanceo/1(Kp_bal)  "Kp_bal"
  MATLAB Function/2(Kd) -> Control PD Balanceo/2(Kd_bal)  "Kd_bal"
  theta/1 -> Control PD Balanceo/3(theta)
  Control PD Balanceo/1(d_x_t*) -> Switch4/1
  Switch4/1 -> Sum/1
  x_td/1 -> Control PID Carro/1(x_td)
  Integrator1/1 -> x_hd*/1, Control PID Izaje/2(x_hd*)
  [x_hd] -> Control PID Izaje/1(x_hd)
  Switch2/1 -> d_x_hd*/1, Integrator1/1
  Control PID Carro/1(T_tm) -> Subsystem2/1(T_tm), T_tm/1
  Integrator/1 -> x_td*/1, Control PID Carro/2(x_td*)
  Switch3/1 -> d_x_td*/1, Integrator/1
  Control PID Izaje/1(T_hm) -> T_hm/1, Subsystem1/1(T_tm)
  Subsystem1/1(T_tm_on) -> T_hm_on/1
  Subsystem2/1(T_tm_on) -> T_tm_on/1

== system modelo_fisico_v18/Subsystem ==
  " " : Inport
  AND : Logic  IconShape=distinctive  AllPortsSameDT=off  OutDataTypeStr=boolean
  BTN_RESET_PRESSED : Constant  Value=0
  Out1 : Outport
  wires:
  BTN_RESET_PRESSED/1 -> AND/2
  " "/1 -> AND/1
  AND/1 -> Out1/1

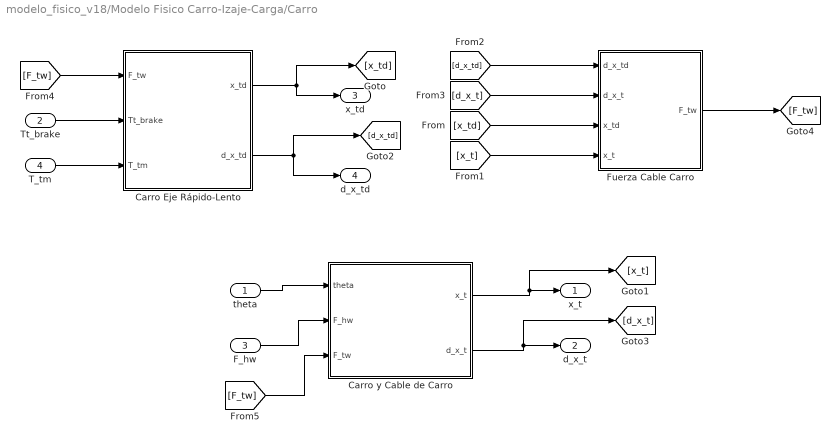
== system modelo_fisico_v18/Modelo Fisico Carro-Izaje-Carga/Carro ==
  theta : Inport
  Tt_brake : Inport  Port=2
  F_hw : Inport  Port=3
  T_tm : Inport  Port=4
  Carro Eje Rápido-Lento : Subsystem
  Carro y Cable de Carro : Subsystem
  Fuerza Cable Carro : Subsystem
  x_t : Outport
  d_x_t : Outport  Port=2
  x_td : Outport  Port=3
  d_x_td : Outport  Port=4
  wires:
  Tt_brake/1 -> Carro Eje Rápido-Lento/2(Tt_brake)
  theta/1 -> Carro y Cable de Carro/1(theta)
  Carro Eje Rápido-Lento/1(x_td) -> x_td/1, [x_td]
  Carro y Cable de Carro/2(d_x_t) -> [d_x_t], d_x_t/1
  Carro Eje Rápido-Lento/2(d_x_td) -> [d_x_td], d_x_td/1
  F_hw/1 -> Carro y Cable de Carro/2(F_hw)
  Carro y Cable de Carro/1(x_t) -> [x_t], x_t/1
  T_tm/1 -> Carro Eje Rápido-Lento/3(T_tm)
  [x_td] -> Fuerza Cable Carro/3(x_td)
  [x_t] -> Fuerza Cable Carro/4(x_t)
  Fuerza Cable Carro/1(F_tw) -> [F_tw]
  [d_x_td] -> Fuerza Cable Carro/1(d_x_td)
  [d_x_t] -> Fuerza Cable Carro/2(d_x_t)
  [F_tw] -> Carro Eje Rápido-Lento/1(F_tw)
  [F_tw] -> Carro y Cable de Carro/3(F_tw)

== system modelo_fisico_v18/Modelo Fisico Carro-Izaje-Carga/Frenos ==
  BRK_t : Inport
  BRK_h : Inport  Port=2
  BRK_hE : Inport  Port=3
  w_tm : Inport  Port=4
  w_hm : Inport  Port=5
  w_hd : Inport  Port=6
  Freno Emergencia Izaje : Subsystem
  Freno Operacion Carro : Subsystem
  Freno Operacion Izaje : Subsystem
  Th_EB : Outport
  Th_brake : Outport  Port=2
  Tt_brake : Outport  Port=3
  wires:
  Freno Operacion Izaje/1(Thb) -> Th_brake/1
  BRK_h/1 -> Freno Operacion Izaje/1(Energizado/Desenergizado)
  BRK_t/1 -> Freno Operacion Carro/1(Energizado/Desenergizado)
  Freno Operacion Carro/1(Ttb) -> Tt_brake/1
  BRK_hE/1 -> Freno Emergencia Izaje/1(Energizado/Desenergizado)
  Freno Emergencia Izaje/1(Th_EB) -> Th_EB/1
  w_tm/1 -> Freno Operacion Carro/2(w_tm)
  w_hm/1 -> Freno Operacion Izaje/2(w_hm)
  w_hd/1 -> Freno Emergencia Izaje/2(w_hd)

== system modelo_fisico_v18/Modelo Fisico Carro-Izaje-Carga/Izaje ==
  l : Inport
  d_l : Inport  Port=2
  T_hm : Inport  Port=3
  T_hEB : Inport  Port=4
  T_hb : Inport  Port=5
  Fuerza cable de Izaje : Subsystem
  Izaje Eje Rapido-Lento : Subsystem
  x_hd : Outport
  d_x_hd : Outport  Port=2
  F_hw : Outport  Port=3
  Tension_hw : Outport  Port=4
  wires:
  T_hb/1 -> Izaje Eje Rapido-Lento/4(T_hb)
  T_hEB/1 -> Izaje Eje Rapido-Lento/3(T_hEb)
  [F_hw] -> Izaje Eje Rapido-Lento/1(F_hw)
  T_hm/1 -> Izaje Eje Rapido-Lento/2(T_hm)
  Fuerza cable de Izaje/1(F_hw) -> [F_hw], F_hw/1
  d_l/1 -> Fuerza cable de Izaje/3(d_l)
  Izaje Eje Rapido-Lento/1(l_h) -> [l_h]
  Izaje Eje Rapido-Lento/3(x_hd) -> x_hd/1
  l/1 -> Fuerza cable de Izaje/1(l)
  Izaje Eje Rapido-Lento/4(d_x_hd) -> d_x_hd/1
  [l_h] -> Fuerza cable de Izaje/2(l_h)
  Izaje Eje Rapido-Lento/2(d_l_h) -> [d_l_h]
  [d_l_h] -> Fuerza cable de Izaje/4(d_l_h)
  Fuerza cable de Izaje/2(Tension_hw) -> Tension_hw/1

== system modelo_fisico_v18/Modelo Fisico Carro-Izaje-Carga/Limites de operacion ==
  vel_hMax : Inport
  x_t : Inport  Port=2
  x_h : Inport  Port=3
  d_x_h : Inport  Port=4
  Límites de Carro : Subsystem
  Subsystem1 : Subsystem
  fc_izq_norm : Outport
  fc_izq_ult : Outport  Port=2
  fc_der_norm : Outport  Port=3
  fc_der_ult : Outport  Port=4
  fc_inf_norm : Outport  Port=5
  fc_inf_ult : Outport  Port=6
  fc_sup_norm : Outport  Port=7
  fc_sup_ult : Outport  Port=8
  lim_v_h : Outport  Port=9
  wires:
  x_t/1 -> Límites de Carro/1(x_t)
  Límites de Carro/1(fc_izq_norm) -> fc_izq_norm/1
  Límites de Carro/2(fc_izq_ult) -> fc_izq_ult/1
  Límites de Carro/3(fc_der_norm) -> fc_der_norm/1
  Límites de Carro/4(fc_der_ult) -> fc_der_ult/1
  Subsystem1/4(fc_sup_ult) -> fc_sup_ult/1
  Subsystem1/3(fc_sup_norm) -> fc_sup_norm/1
  Subsystem1/2(fc_inf_ult) -> fc_inf_ult/1
  Subsystem1/1(fc_inf_norm) -> fc_inf_norm/1
  x_h/1 -> Subsystem1/1(x_h)
  d_x_h/1 -> Subsystem1/3(d_x_h)
  Subsystem1/5(lim_v_h) -> lim_v_h/1
  vel_hMax/1 -> Subsystem1/2(vel_hMax)

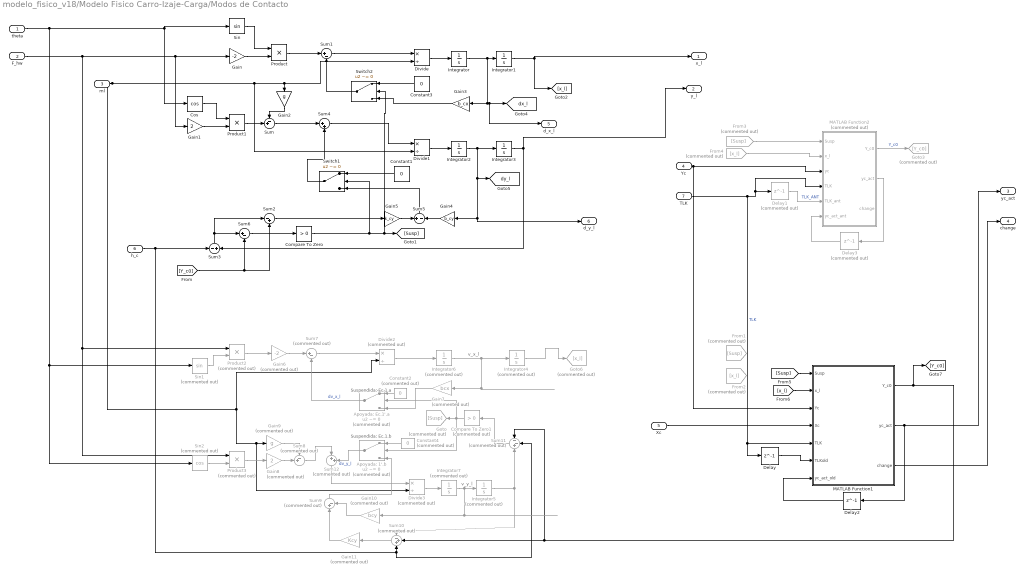
== system modelo_fisico_v18/Modelo Fisico Carro-Izaje-Carga/Modos de Contacto ==
  note: v_y_l
  note: v_x_l
  note: Suspendida: Ec.1.a
  note: Suspendida: Ec.1.b
  theta : Inport
  F_hw : Inport  Port=2
  ml : Inport  Port=3
  Yc : Inport  Port=4
  Xc : Inport  Port=5
  h_c : Inport  Port=6
  TLK : Inport  Port=7
  Apoyada: 1'.b : Switch  Commented=on  Criteria=u2 ~= 0
  Apoyada: Ec.1'.a : Switch  Commented=on  Criteria=u2 ~= 0
  Compare To Zero : simulink/Logic and Bit Operations/Compare To Zero  relop=>  OutDataTypeStr=boolean
  Compare To Zero1 : simulink/Logic and Bit Operations/Compare To Zero  Commented=on  relop=>  OutDataTypeStr=boolean
  Constant1 : Constant  Value=0
  Constant2 : Constant  Commented=on  Value=0
  Constant3 : Constant  Value=0
  Constant4 : Constant  Commented=on  Value=0
  Cos : Trigonometry  Operator=cos
  Delay : Delay  DelayLength=1
  Delay1 : Delay  Commented=on  DelayLength=1
  Delay2 : Delay  DelayLength=1
  Delay3 : Delay  Commented=on  DelayLength=1
  Divide : Product  Inputs=*/
  Divide1 : Product  Inputs=*/
  Divide2 : Product  Commented=on  Inputs=*/
  Divide3 : Product  Commented=on  Inputs=*/
  From1 : From  Commented=on  GotoTag=Susp
  From2 : From  Commented=on  GotoTag=x_l
  From3 : From  Commented=on  GotoTag=Susp
  From4 : From  Commented=on  GotoTag=x_l
  Gain : Gain  Gain=-2
  Gain1 : Gain  Gain=2
  Gain10 : Gain  Commented=on  Gain=bcy
  Gain11 : Gain  Commented=on  Gain=Kcy
  Gain2 : Gain  Gain=g
  Gain3 : Gain  Gain=b_cx
  Gain4 : Gain  Gain=b_cy
  Gain5 : Gain  Gain=k_cy
  Gain6 : Gain  Commented=on  Gain=-2
  Gain7 : Gain  Commented=on  Gain=bcx
  Gain8 : Gain  Commented=on  Gain=2
  Gain9 : Gain  Commented=on  Gain=g
  Goto : Goto  Commented=on  GotoTag=Susp
  Goto3 : Goto  Commented=on  GotoTag=Y_c0
  Goto6 : Goto  Commented=on  GotoTag=x_l
  Integrator : Integrator
  Integrator1 : Integrator  InitialCondition=CI_t
  Integrator2 : Integrator
  Integrator3 : Integrator  InitialCondition=CI_h
  Integrator4 : Integrator  Commented=on  InitialCondition=Cond_Ini_t
  Integrator5 : Integrator  Commented=on  InitialCondition=Cond_Ini_h
  Integrator6 : Integrator  Commented=on
  Integrator7 : Integrator  Commented=on
  MATLAB Function1 : MATLAB Function  TreatAsAtomicUnit=on
  MATLAB Function2 : MATLAB Function  Commented=on  TreatAsAtomicUnit=on
  Product : Product
  Product1 : Product
  Product2 : Product  Commented=on
  Product3 : Product  Commented=on
  Sin : Trigonometry
  Sin1 : Trigonometry  Commented=on
  Sin2 : Trigonometry  Commented=on  Operator=cos
  Sum : Sum  Inputs=-+|
  Sum1 : Sum  Inputs=|+-
  Sum10 : Sum  Commented=on  Inputs=-++
  Sum11 : Sum  Commented=on  Inputs=--+
  Sum12 : Sum  Commented=on  Inputs=|++
  Sum2 : Sum  Inputs=|-+
  Sum3 : Sum  Inputs=-|+
  Sum4 : Sum  Inputs=|++
  Sum5 : Sum  Inputs=+|-
  Sum6 : Sum  Inputs=|+-
  Sum7 : Sum  Commented=on  Inputs=|+-
  Sum8 : Sum  Commented=on  Inputs=-+|
  Sum9 : Sum  Commented=on  Inputs=|+-
  Switch1 : Switch  Criteria=u2 ~= 0
  Switch2 : Switch  Criteria=u2 ~= 0
  x_l : Outport
  y_l : Outport  Port=2
  yc_act : Outport  Port=3
  change : Outport  Port=4
  d_x_l : Outport  Port=5
  d_y_l : Outport  Port=6
  tag scope: dx_l=global, dy_l=global
  wires:
  Gain/1 -> Product/2
  Sin/1 -> Product/1
  Cos/1 -> Product1/1
  Gain1/1 -> Product1/2
  Divide/1 -> Integrator/1
  Integrator/1 -> Integrator1/1, d_x_l/1, [dx_l], Gain3/1
  Divide1/1 -> Integrator2/1
  Integrator2/1 -> [dy_l], d_y_l/1, Gain4/1, Integrator3/1
  Integrator3/1 -> Sum3/2, y_l/1
  Product/1 -> Sum1/1
  Sum1/1 -> Divide/1
  Switch2/1 -> Sum1/2
  Constant3/1 -> Switch2/1
  Gain3/1 -> Switch2/3
  Sum5/1 -> Switch1/3
  Gain5/1 -> Sum5/1
  Gain4/1 -> Sum5/2
  Constant1/1 -> Switch1/1
  h_c/1 -> Sum3/1, Sum11/2, Sum10/3
  Sum3/1 -> Sum6/1, Sum2/1
  Sum/1 -> Sum4/1
  Sum4/1 -> Divide1/1
  Switch1/1 -> Sum4/2
  Product1/1 -> Sum/2
  Gain2/1 -> Sum/1
  Integrator1/1 -> [x_l], x_l/1
  Sum2/1 -> Gain5/1
  Sum6/1 -> Compare To Zero/1
  F_hw/1 -> Product3/1, Product2/1, Gain/1, Gain1/1
  Compare To Zero/1 -> [Susp], Switch2/2, Switch1/2
  From4/1 -> MATLAB Function2/2(x_l)
  MATLAB Function2/1(Y_c0) -> Goto3/1  "Y_c0"
  MATLAB Function2/2(yc_act) -> Delay3/1
  From3/1 -> MATLAB Function2/1(Susp)
  Delay1/1 -> MATLAB Function2/5(TLK_ant)  "TLK_ANT"
  TLK/1 -> Delay/1, MATLAB Function1/5(TLK), MATLAB Function2/4(TLK), Delay1/1  "TLK"
  Delay3/1 -> MATLAB Function2/6(yc_act_ant)
  Sum8/1 -> Sum12/1
  Constant2/1 -> Apoyada: Ec.1'.a/1
  Divide3/1 -> Integrator7/1
  Gain6/1 -> Sum7/1
  Sin2/1 -> Product3/2
  Yc/1 -> MATLAB Function2/3(yc), MATLAB Function1/3(Yc)
  Xc/1 -> MATLAB Function1/4(Xc)
  Sum7/1 -> Divide2/1
  ml/1 -> Divide/2, Gain2/1, Divide1/2, Divide2/2, Divide3/2, Gain9/1
  MATLAB Function1/2(yc_act) -> yc_act/1, Delay2/1
  MATLAB Function1/3(change) -> change/1
  Delay2/1 -> MATLAB Function1/7(yc_act_old)
  Sin1/1 -> Product2/2
  [x_l] -> MATLAB Function1/2(x_l)
  [Susp] -> MATLAB Function1/1(Susp)
  MATLAB Function1/1(Y_c0) -> [Y_c0], Sum10/2, Sum11/1
  Delay/1 -> MATLAB Function1/6(TLKold)
  Sum11/1 -> Compare To Zero1/1
  Sum10/1 -> Gain11/1
  Integrator6/1 -> Gain7/1, Integrator4/1
  Gain8/1 -> Sum8/2
  Gain9/1 -> Sum8/1
  Product2/1 -> Gain6/1
  Product3/1 -> Gain8/1
  Apoyada: Ec.1'.a/1 -> Sum7/2  "dv_x_l"
  Divide2/1 -> Integrator6/1
  theta/1 -> Sin2/1, Sin1/1, Sin/1, Cos/1
  Sum12/1 -> Divide3/1
  Compare To Zero1/1 -> Goto/1, Apoyada: Ec.1'.a/2, Apoyada: 1'.b/2
  Sum9/1 -> Apoyada: 1'.b/3
  Gain7/1 -> Apoyada: Ec.1'.a/3
  Gain10/1 -> Sum9/2
  Gain11/1 -> Sum9/1
  Integrator7/1 -> Gain10/1, Integrator5/1
  Constant4/1 -> Apoyada: 1'.b/1
  Integrator5/1 -> Sum11/3, Sum10/1
  Apoyada: 1'.b/1 -> Sum12/2  "dv_y_l"
  Integrator4/1 -> Goto6/1
  [Y_c0] -> Sum2/2, Sum6/2

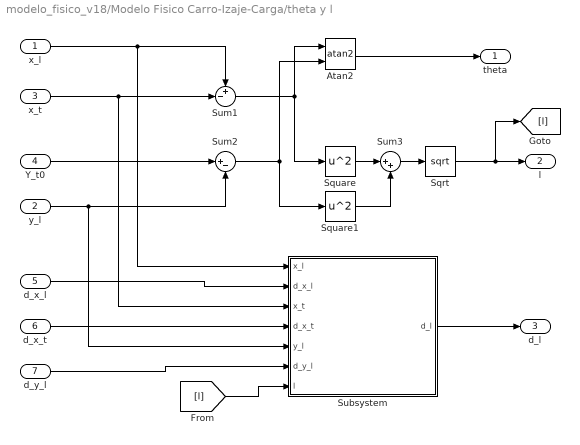
== system modelo_fisico_v18/Modelo Fisico Carro-Izaje-Carga/theta y l ==
  x_l : Inport
  y_l : Inport  Port=2
  x_t : Inport  Port=3
  Y_t0 : Inport  Port=4
  d_x_l : Inport  Port=5
  d_x_t : Inport  Port=6
  d_y_l : Inport  Port=7
  Atan2 : Trigonometry  Operator=atan2
  Sqrt : Sqrt  SaturateOnIntegerOverflow=on
  Square : Math  Operator=square  SaturateOnIntegerOverflow=on
  Square1 : Math  Operator=square  SaturateOnIntegerOverflow=on
  Subsystem : Subsystem
  Sum1 : Sum  Inputs=+-|
  Sum2 : Sum  Inputs=|+-
  Sum3 : Sum  Inputs=|++
  theta : Outport
  l : Outport  Port=2
  d_l : Outport  Port=3
  wires:
  x_l/1 -> Subsystem/1(x_l), Sum1/1
  x_t/1 -> Subsystem/3(x_t), Sum1/2
  Y_t0/1 -> Sum2/1
  y_l/1 -> Subsystem/5(y_l), Sum2/2
  Sum1/1 -> Square/1, Atan2/1
  Sum2/1 -> Square1/1, Atan2/2
  Sum3/1 -> Sqrt/1
  Sqrt/1 -> [l], l/1
  Square/1 -> Sum3/1
  Square1/1 -> Sum3/2
  Atan2/1 -> theta/1
  [l] -> Subsystem/7(l)
  d_x_l/1 -> Subsystem/2(d_x_l)
  d_x_t/1 -> Subsystem/4(d_x_t)
  d_y_l/1 -> Subsystem/6(d_y_l)
  Subsystem/1(d_l) -> d_l/1

== system modelo_fisico_v18/Nivel 2/Control PD Balanceo ==
  Kp_bal : Inport
  Kd_bal : Inport  Port=2
  theta : Inport  Port=3
  Constant2 : Constant  Value=0
  Delay One Step : Delay  DelayLength=1  SampleTime=1e-3
  Gain1 : Gain  Gain=1/1e-3
  Product : Product
  Product1 : Product
  Sum1 : Sum  Inputs=|+-
  Sum2 : Sum  Inputs=|+-
  Sum3 : Sum  Inputs=|++
  d_x_t* : Outport
  wires:
  Product1/1 -> Sum3/1
  Gain1/1 -> Product/2
  Kp_bal/1 -> Product1/1
  Product/1 -> Sum3/2
  Sum2/1 -> Gain1/1
  Constant2/1 -> Sum1/1
  Sum1/1 -> Product1/2, Sum2/1, Delay One Step/1
  Delay One Step/1 -> Sum2/2
  theta/1 -> Sum1/2
  Kd_bal/1 -> Product/1
  Sum3/1 -> d_x_t*/1

== system modelo_fisico_v18/Nivel 2/Control PID Carro ==
  x_td : Inport
  x_td* : Inport  Port=2
  Gain : Gain  Gain=1/tau_tm
  Integrator : Integrator  InitialConditionSource=external
  PID Traslacion : Subsystem
  Sum : Sum  Inputs=|+-
  T_tmMax : Saturate  UpperLimit=T_tmMax  LowerLimit=-T_tmMax
  T_tm : Outport
  wires:
  PID Traslacion/1(T_tm*) -> T_tmMax/1
  x_td*/1 -> PID Traslacion/1(x_td*)
  x_td/1 -> PID Traslacion/2(x_td)
  T_tmMax/1 -> Integrator/2, Sum/1
  Sum/1 -> Gain/1
  Gain/1 -> Integrator/1
  Integrator/1 -> T_tm/1, Sum/2

== system modelo_fisico_v18/Nivel 2/Control PID Izaje ==
  x_hd : Inport
  x_hd* : Inport  Port=2
  Gain : Gain  Gain=1/tau_hm
  Integrator : Integrator  InitialConditionSource=external
  PID Izaje : Subsystem
  Saturation1 : Saturate  UpperLimit=T_hmMax  LowerLimit=-T_hmMax
  Sum : Sum  Inputs=|+-
  T_hm : Outport
  wires:
  PID Izaje/1(T_hm) -> Saturation1/1
  x_hd*/1 -> PID Izaje/1(x_h*)
  x_hd/1 -> PID Izaje/2(x_h)
  Gain/1 -> Integrator/1
  Sum/1 -> Gain/1
  Saturation1/1 -> Integrator/2, Sum/1
  Integrator/1 -> T_hm/1, Sum/2

== system modelo_fisico_v18/Nivel 2/Subsystem1 ==
  T_tm : Inport
  AND : Logic  Operator=NAND  Inputs=3  IconShape=distinctive  AllPortsSameDT=off  OutDataTypeStr=boolean
  Abs1 : Abs
  Abs2 : Abs
  Abs3 : Abs
  Compare To Constant1 : simulink/Logic and Bit Operations/Compare To Constant  relop=<  const=1e-3  OutDataTypeStr=boolean
  Compare To Constant2 : simulink/Logic and Bit Operations/Compare To Constant  relop=<  const=1e-3  OutDataTypeStr=boolean
  Compare To Constant3 : simulink/Logic and Bit Operations/Compare To Constant  relop=<  const=1e-3  OutDataTypeStr=boolean
  Memory : Memory
  Memory1 : Memory
  T_tm_on : Outport
  wires:
  Abs1/1 -> Compare To Constant1/1
  T_tm/1 -> Abs1/1, Memory/1
  Abs2/1 -> Compare To Constant2/1
  Memory/1 -> Abs2/1, Memory1/1
  Abs3/1 -> Compare To Constant3/1
  Memory1/1 -> Abs3/1
  Compare To Constant1/1 -> AND/1
  Compare To Constant2/1 -> AND/2
  Compare To Constant3/1 -> AND/3
  AND/1 -> T_tm_on/1

== system modelo_fisico_v18/Nivel 2/Subsystem2 ==
  T_tm : Inport
  AND : Logic  Operator=NAND  Inputs=3  IconShape=distinctive  AllPortsSameDT=off  OutDataTypeStr=boolean
  Abs1 : Abs
  Abs2 : Abs
  Abs3 : Abs
  Compare To Constant1 : simulink/Logic and Bit Operations/Compare To Constant  relop=<  const=1e-3  OutDataTypeStr=boolean
  Compare To Constant2 : simulink/Logic and Bit Operations/Compare To Constant  relop=<  const=1e-3  OutDataTypeStr=boolean
  Compare To Constant3 : simulink/Logic and Bit Operations/Compare To Constant  relop=<  const=1e-3  OutDataTypeStr=boolean
  Memory : Memory
  Memory1 : Memory
  T_tm_on : Outport
  wires:
  Abs1/1 -> Compare To Constant1/1
  T_tm/1 -> Abs1/1, Memory/1
  Abs2/1 -> Compare To Constant2/1
  Memory/1 -> Abs2/1, Memory1/1
  Abs3/1 -> Compare To Constant3/1
  Memory1/1 -> Abs3/1
  Compare To Constant1/1 -> AND/1
  Compare To Constant2/1 -> AND/2
  Compare To Constant3/1 -> AND/3
  AND/1 -> T_tm_on/1

== system modelo_fisico_v18/Modelo Fisico Carro-Izaje-Carga/Carro/Carro Eje Rápido-Lento ==
  F_tw : Inport
  Tt_brake : Inport  Port=2
  T_tm : Inport  Port=3
  1/Meq_t : Gain  Gain=1/M_eq_t
  Gain3 : Gain  Gain=i_t/r_td
  Integrator2 : Integrator
  Integrator3 : Integrator  InitialCondition=CI_t
  Sum : Sum  Inputs=|++
  Sum1 : Sum  Inputs=-+-
  beq_t : Gain  Gain=b_eq_t
  x_td : Outport
  d_x_td : Outport  Port=2
  wires:
  Integrator2/1 -> d_x_td/1, beq_t/1, Integrator3/1
  Integrator3/1 -> x_td/1
  1/Meq_t/1 -> Integrator2/1
  Sum1/1 -> 1/Meq_t/1
  beq_t/1 -> Sum1/3
  F_tw/1 -> Sum1/1
  T_tm/1 -> Sum/1  "Tmotor"
  Tt_brake/1 -> Sum/2  "Tt_brake"
  Sum/1 -> Gain3/1
  Gain3/1 -> Sum1/2

== system modelo_fisico_v18/Modelo Fisico Carro-Izaje-Carga/Carro/Carro y Cable de Carro ==
  theta : Inport
  F_hw : Inport  Port=2
  F_tw : Inport  Port=3
  1/M_t : Gain  Gain=1/M_t
  Gain : Gain  Gain=2
  Integrator : Integrator  InitialCondition=CI_t
  Integrator2 : Integrator
  Product : Product
  Sin : Trigonometry
  Sum1 : Sum  Inputs=++-
  b_t : Gain  Gain=b_t
  x_t : Outport
  d_x_t : Outport  Port=2
  wires:
  Sum1/1 -> 1/M_t/1
  Integrator2/1 -> d_x_t/1, b_t/1, Integrator/1
  theta/1 -> Sin/1
  Sin/1 -> Product/2
  F_hw/1 -> Gain/1
  Gain/1 -> Product/1
  Product/1 -> Sum1/2
  b_t/1 -> Sum1/3
  1/M_t/1 -> Integrator2/1
  Integrator/1 -> x_t/1
  F_tw/1 -> Sum1/1

== system modelo_fisico_v18/Modelo Fisico Carro-Izaje-Carga/Carro/Fuerza Cable Carro ==
  d_x_td : Inport
  d_x_t : Inport  Port=2
  x_td : Inport  Port=3
  x_t : Inport  Port=4
  Gain : Gain  Gain=k_tw
  Gain1 : Gain  Gain=b_tw
  Sum : Sum  Inputs=+|-
  Sum1 : Sum  Inputs=+|-
  Sum2 : Sum  Inputs=+|+
  F_tw : Outport
  wires:
  x_td/1 -> Sum/1
  Gain/1 -> Sum2/2
  Gain1/1 -> Sum2/1
  d_x_td/1 -> Sum1/1
  x_t/1 -> Sum/2
  Sum1/1 -> Gain1/1
  Sum2/1 -> F_tw/1
  Sum/1 -> Gain/1
  d_x_t/1 -> Sum1/2

== system modelo_fisico_v18/Modelo Fisico Carro-Izaje-Carga/Frenos/Freno Emergencia Izaje ==
  Energizado/Desenergizado : Inport
  w_hd : Inport  Port=2
  Constant : Constant  Value=0
  Gain : Gain  Gain=-b_hEb
  Saturation : Saturate  UpperLimit=T_hEbMax  LowerLimit=-T_hEbMax
  Switch : Switch  Criteria=u2 ~= 0
  Th_EB : Outport
  wires:
  Energizado/Desenergizado/1 -> Switch/2
  Constant/1 -> Switch/1
  w_hd/1 -> Gain/1
  Gain/1 -> Saturation/1
  Saturation/1 -> Switch/3
  Switch/1 -> Th_EB/1

== system modelo_fisico_v18/Modelo Fisico Carro-Izaje-Carga/Frenos/Freno Operacion Carro ==
  Energizado/Desenergizado : Inport
  w_tm : Inport  Port=2
  Constant : Constant  Value=0
  Gain : Gain  Gain=-b_tb
  Saturation : Saturate  UpperLimit=T_tbMax  LowerLimit=-T_tbMax
  Switch : Switch  Criteria=u2 ~= 0
  Ttb : Outport
  wires:
  Energizado/Desenergizado/1 -> Switch/2
  Constant/1 -> Switch/1
  w_tm/1 -> Gain/1
  Gain/1 -> Saturation/1
  Saturation/1 -> Switch/3
  Switch/1 -> Ttb/1

== system modelo_fisico_v18/Modelo Fisico Carro-Izaje-Carga/Frenos/Freno Operacion Izaje ==
  Energizado/Desenergizado : Inport
  w_hm : Inport  Port=2
  Constant : Constant  Value=0
  Gain : Gain  Gain=-b_hb
  Saturation : Saturate  UpperLimit=T_hbMax  LowerLimit=-T_hbMax
  Switch : Switch  Criteria=u2 ~= 0
  Thb : Outport
  wires:
  Energizado/Desenergizado/1 -> Switch/2
  Constant/1 -> Switch/1
  w_hm/1 -> Gain/1
  Gain/1 -> Saturation/1
  Saturation/1 -> Switch/3
  Switch/1 -> Thb/1
